simulink model "Proj_5_part_3"  (R2017a)
settings: Solver=ode4  StartTime=0.0  StopTime=1370  FixedStep=0.001  RelTol=1e-3
undefined symbols (not defined in the file or in its folder): t_city_cycle, v_city_cycle
settings Model: Creator=apple  LastModifiedBy=Jinesh

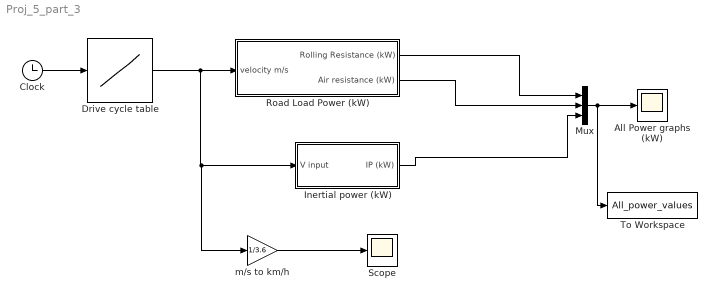
== system Proj_5_part_3 ==
  All Power graphs (kW) : Scope
  Clock : Clock
  Drive cycle table : Lookup_n-D  NumberOfTableDimensions=1  BreakpointsForDimension1=t_city_cycle  Table=v_city_cycle  InternalRulePriority=Speed  RndMeth=Simplest  InputSameDT=on
  Inertial power (kW) : Subsystem  TreatAsAtomicUnit=on
  Mux : Mux  Inputs=3
  Road Load Power (kW) : Subsystem  TreatAsAtomicUnit=on
  Scope : Scope
  To Workspace : ToWorkspace  VariableName=All_power_values  SaveFormat=Timeseries  SampleTime=-1
  m/s to km/h : Gain  Gain=1/3.6
  wires:
  Inertial power (kW)/1(IP (kW)) -> Mux/3
  m/s to km/h/1 -> Scope/1
  Drive cycle table/1 -> m/s to km/h/1, Inertial power (kW)/1(V input), Road Load Power (kW)/1("velocity m/s ")
  Mux/1 -> To Workspace/1, All Power graphs (kW)/1
  Road Load Power (kW)/2(Air resistance (kW)) -> Mux/2
  Road Load Power (kW)/1(Rolling Resistance (kW)) -> Mux/1
  Clock/1 -> Drive cycle table/1

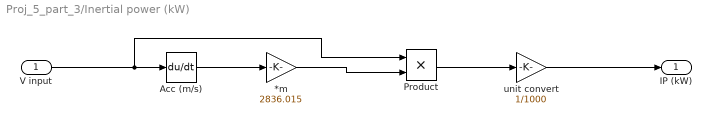
== system Proj_5_part_3/Inertial power (kW) ==
  V input : Inport
  *m : Gain  Gain=2836.015
  Acc (m/s) : Derivative
  Product : Product
  unit convert : Gain  Gain=1/1000
  IP (kW) : Outport
  wires:
  V input/1 -> Product/1, Acc (m/s)/1
  Acc (m/s)/1 -> *m/1
  *m/1 -> Product/2
  Product/1 -> unit convert/1
  unit convert/1 -> IP (kW)/1

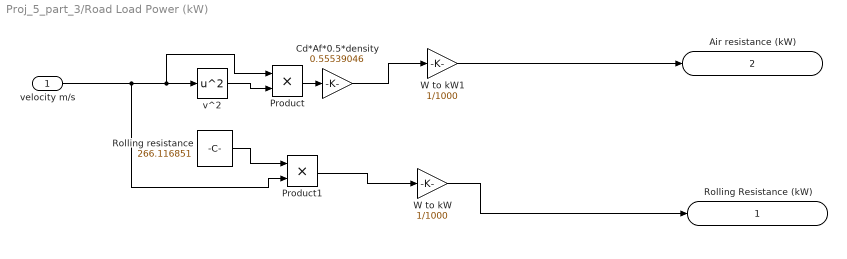
== system Proj_5_part_3/Road Load Power (kW) ==
  "velocity m/s " : Inport
  "Cd*Af*0.5*density " : Gain  Gain=0.55539046
  Product : Product
  Product1 : Product
  "Rolling resistance " : Constant  Value=266.116851
  W to kW : Gain  Gain=1/1000
  W to kW1 : Gain  Gain=1/1000
  v^2 : Math  Operator=square  SaturateOnIntegerOverflow=on
  Rolling Resistance (kW) : Outport
  Air resistance (kW) : Outport  Port=2
  wires:
  "velocity m/s "/1 -> Product1/2, Product/1, v^2/1
  Product/1 -> "Cd*Af*0.5*density "/1
  v^2/1 -> Product/2
  "Rolling resistance "/1 -> Product1/1
  "Cd*Af*0.5*density "/1 -> W to kW1/1
  W to kW1/1 -> Air resistance (kW)/1
  Product1/1 -> W to kW/1
  W to kW/1 -> Rolling Resistance (kW)/1
